simulink model "sl_pursuit_unicycle"  (R2023a)
settings: Solver=ode45  StartTime=0.0  StopTime=76  FixedStep=0.2  MaxStep=0.1  RelTol=1e-3  EnableMultiTasking=on
StartFcn:
  | % remove the red dashed line draw in StopFcn
  | h = findobj('Tag',  'SL_PURSUIT_PATH');
  | if ~isempty(h)
  |     delete(h)
  | end
StopFcn:
  | % get the waypoints from trajectory block
  | h = getSimulinkBlockHandle([gcs '/trajectory'])
  | path = str2num(get_param(h, 'path'));
  | 
  | % overlay it on the XY scope, tag it so it can be cleaned up in StartFcn
  | set(0, 'ShowHiddenHandles', 'on')
  | fig = findobj('name', 'XY');
  | ax = findobj('type', 'axes');
  | axes(ax);
  | hold on
  | plot(path(:,1), path(:,2), 'Color',  'red', 'LineStyle', '--', 'LineWidth', 2, 'Tag', 'SL_PURSUIT_PATH')
  | grid on
  | hold off
  | set(0, 'ShowHiddenHandles', 'on')
libraries: roblocks x2, simulink_need_slupdate x1
settings Model: Creator=pic  LastModifiedBy=bmake
settings SolverCC: AlgebraicLoopSolver=TrustRegion
settings DataIOCC: SaveFormat=Array  SignalLoggingSaveFormat=ModelDataLogs  TimeSaveName=t  OutputSaveName=y
settings OptimizationCC: ExpressionDepthLimit=2147483647  LifeSpan=inf
settings DebuggingCC: UnderspecifiedInitializationDetection=Classic  MergeDetectMultiDrivingBlocksExec=none  SolverPrmCheckMsg=warning  FcnCallInpInsideContextMsg=warning  UnconnectedInputMsg=warning  UnconnectedOutputMsg=warning  UnconnectedLineMsg=warning  AllowSymbolicDim=off  StateNameClashWarn=warning  SFUnexpectedBacktrackingDiag=warning  SFNoUnconditionalDefaultTransitionDiag=warning  SFExecutionAtInitializationDiag=none  ArithmeticOperatorsInVariantConditions=warning
settings HardwareCC: ProdBitPerPointer=32  ProdBitPerSizeT=32  ProdBitPerPtrDiffT=32  ProdLargestAtomicFloat=None  ProdIntDivRoundTo=Undefined  ProdEndianess=Unspecified  ProdWordSize=32  ProdHWDeviceType=32-bit Generic
settings ModelReferenceCC: EnableRefExpFcnMdlSchedulingChecks=on  PropagateSignalLabelsOutOfModel=off
settings SFSimCC: SimUseLocalCustomCode=off  CustomCodeUndefinedFunction=UseInterfaceOnly
settings RTWCC: RTWUseLocalCustomCode=off
settings CodeAppCC: StateflowObjectComments=on
settings GRTTargetCC: TargetLangStandard=C89/C90 (ANSI)  CombineOutputUpdateFcns=off  GRTInterface=on
settings ConfigComp: CovMetricSettings=dw  CovSaveCumulativeToWorkspaceVar=on  CovSaveSingleToWorkspaceVar=on  CovExternalEMLEnable=off

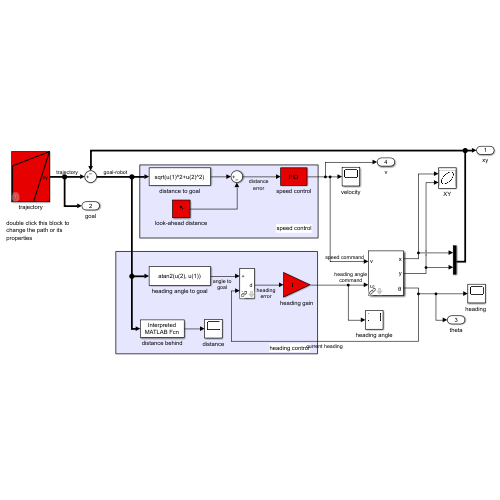
[thumbnail: Simulink's stored preview of the top-level diagram]
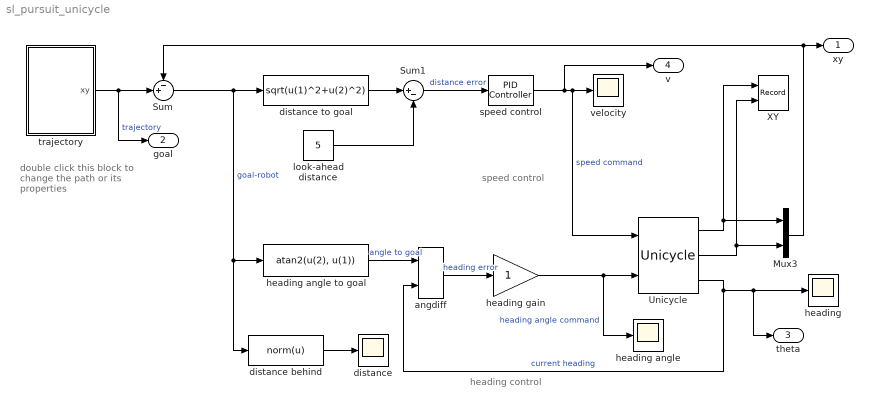
== system sl_pursuit_unicycle ==
  note: speed control
  note: heading control
  note: double click this block to
      | change the path or its
      | properties
  Mux3 : Mux  Inputs=2
  Sum : Sum  Inputs=-+|
  Sum1 : Sum  Inputs=|+-
  Unicycle : roblocks/Vehicles/Unicycle  alim=1  vlim=5  wlim=10  x0=[0, 0, 0]  a=0.1
  XY : Record  FileSettingsInternal="{\"entries\":[{\"content\":{\"excelSettings\":{\"content\":{},\"type\":\"Streamout.ExcelSettings\"}},\"type\":\"Streamout.FileSettingStorage\",\"uuid\":\"\"}],\"packageUris\":[\"http:\\/\\/schema.mathworks.com\\/mf0\\/streamout_blocks\\/R2020a\"],\"version\":\"1.0\"}"  Layout=[1 1]  SignalsInternal="{\"entries\":[{\"content\":{\"signals\":[{\"content\":{\"blockPath\":[],\"dimensions\":[1],\"domain\":\"\",\"lineColor\":\"#a2142f\",\"plots\":[1],\"port\":1,\"sid\":[\"\"],\"signalID\":27,\"signalName\":\"Unicycle:1\"},\"type\":\"RecordBlkView.Signal\",\"uuid\":\"\"},{\"content\":{\"blockPath\":[],\"dimensions\":[1],\"domain\":\"\",\"lineColor\":\"#139fff\",\"plots\":[1],\"port\":2,\"sid\":[\"\"],\"signalID\":31,\"signalName\":\"Unicycle:2\"},\"type\":\"RecordBlkView.Signal\",\"uuid\":\"\"}]},\"type\":\"RecordBlkView.InputSignals\",\"uuid\":\"\"}],\"packageUris\":[\"http:\\/\\/schema.mathworks.com\\/mf0\\/streamout_blocks\\/R2020a\"],\"version\":\"1.0\"}"  VisualizationBindings="{\"xyplotplugin\":{\"info\":[{\"series\":[{\"bindingParametersList\":[{\"parameter\":\"X-Axis\",\"signalID\":27,\"signalName\":\"Unicycle:1\"},{\"parameter\":\"Y-Axis\",\"signalID\":31,\"signalName\":\"Unicycle:2\"}],\"seriesID\":6249}],\"subplotID\":1}]}}"  CompatibilityTag=XY  st=-1
  angdiff : roblocks/Toolbox/angdiff
  distance : Scope
  distance behind : MATLABFcn  MATLABFcn=norm(u)
  distance to goal : Fcn  Expr=sqrt(u(1)^2+u(2)^2)
  "heading " : Scope
  heading angle : Scope
  heading angle to goal : Fcn  Expr=atan2(u(2), u(1))
  heading gain : Gain
  look-ahead distance : Constant  Value=5
  speed control : simulink_need_slupdate/PID Controller  P=1  I=0.1  D=0
  trajectory : Subsystem  mask(Trajectory generator){path=|, vaxis=[2.5 2.5], tseg=[], dt=0.1, tacc=0, setsimtime=on}
      mask path=|
      | [  10 10;
      |   10 60;
      |   80 80;
      |   50 10 ]
      mask prompts: vaxis "Axis velocities"; tseg "Segment times"; dt "Sample interval"; tacc "Acceleration time"; setsimtime "Set Simulink simulation time"
      mask help: Generate an n-dimensional trajectory using the Toolbox function mstraj.
      mask init:
      | robot_traj = mstraj(path(2:end,:), vaxis, tseg, path(1,:), dt, tacc);
      | total_time = size(robot_traj,1)*dt;
      | if setsimtime
      |     set_param(gcs, 'StopTime', num2str(total_time));
      | end
      mask Help:
      | The trajectory requires a number of parameters
      | 
      | Path: an MxN matrix that defines a path with M points (start, intermediate, goal) and each point is defined by an N-dimensional vector.
      | 
      | Axis velocities: a 1xM vector that specifies the maximum speed of each motion for each dimension.
      | 
      | Segment times: a 1x(N-1) vector of times to execute each motion segment.
      | 
      | Sample time: a scalar sampling time, the trajectory is computed at discrete times with this separation.
      | 
      | Acceleration time: a scalar giving the period of acceleration at each waypoint, as the motion accelerates from one segment to the next.  Can be zero.
      | 
      | This block sets the Simulink simulation time to the length of the trajectory.
      mask Display: plot(path(:,1), path(:,2))
  velocity : Scope
  xy : Outport  VectorParamsAs1DForOutWhenUnconnected=off
  goal : Outport  Port=2  VectorParamsAs1DForOutWhenUnconnected=off
  theta : Outport  Port=3  VectorParamsAs1DForOutWhenUnconnected=off
  v : Outport  Port=4  VectorParamsAs1DForOutWhenUnconnected=off
  wires:
  Unicycle/1 -> Mux3/1, XY/1
  Unicycle/2 -> XY/2, Mux3/2
  Mux3/1 -> Sum/1, xy/1
  Sum/1 -> distance behind/1, heading angle to goal/1, distance to goal/1  "goal-robot"
  heading angle to goal/1 -> angdiff/1  "angle to goal"
  Unicycle/3 -> "heading "/1, theta/1, angdiff/2  "current heading"
  angdiff/1 -> heading gain/1  "heading error"
  heading gain/1 -> Unicycle/2, heading angle/1  "heading angle command"
  speed control/1 -> Unicycle/1, velocity/1, v/1  "speed command"
  distance behind/1 -> distance/1
  trajectory/1(xy) -> goal/1, Sum/2  "trajectory"
  Sum1/1 -> speed control/1  "distance error"
  look-ahead distance/1 -> Sum1/2
  distance to goal/1 -> Sum1/1

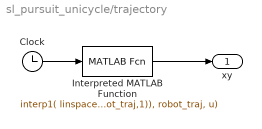
== system sl_pursuit_unicycle/trajectory ==
  Clock : Clock
  Interpreted MATLAB Function : MATLABFcn  MATLABFcn=interp1( linspace(0, total_time, size(robot_traj,1)), robot_traj, u)
  xy : Outport  VectorParamsAs1DForOutWhenUnconnected=off
  wires:
  Clock/1 -> Interpreted MATLAB Function/1
  Interpreted MATLAB Function/1 -> xy/1
